simulink model "test_loadcase_pack_harness"  (R2026a)
settings: Solver=VariableStepAuto  StopTime=2000  AbsTol=1e-3
libraries: fl_lib x3, simulink x2, pack_5p48s8p_Thr_library x2, nesl_utility x2, pack_5p48s8p_1g10g1_5g1g5_Thr_library x1, pack_5p48s8p_1g10g1_Thr_library x1
Description:
  | Copyright 2023-2026 The MathWorks, Inc.
settings Model: Creator=smiller  LastModifiedBy=smiller
settings DebuggingCC: SymbolicDimsDataTypeCodeGenerationDiagnostic=none
settings SimscapeCC: SimscapeNominalValues="[{\"value\":\"1\",\"unit\":\"A\"},{\"value\":\"1\",\"unit\":\"bar\"},{\"value\":\"1\",\"unit\":\"cm^2\"},{\"value\":\"1\",\"unit\":\"cm^3/s\"},{\"value\":\"1\",\"unit\":\"kJ/kg\"},{\"value\":\"1\",\"unit\":\"kW\"},{\"value\":\"1\",\"unit\":\"l\"},{\"value\":\"1\",\"unit\":\"N\"},{\"value\":\"1\",\"unit\":\"N*m\"},{\"value\":\"1\",\"unit\":\"V\"}]"  SimscapeLogSimulationStatistics=on  SimscapeLogName=simlog_test_loadcase_pack

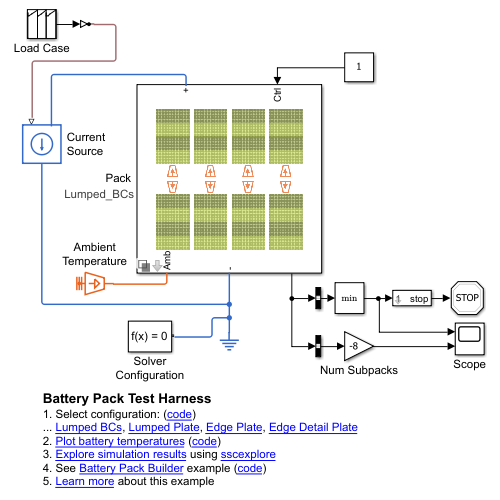
[thumbnail: Simulink's stored preview of the top-level diagram]
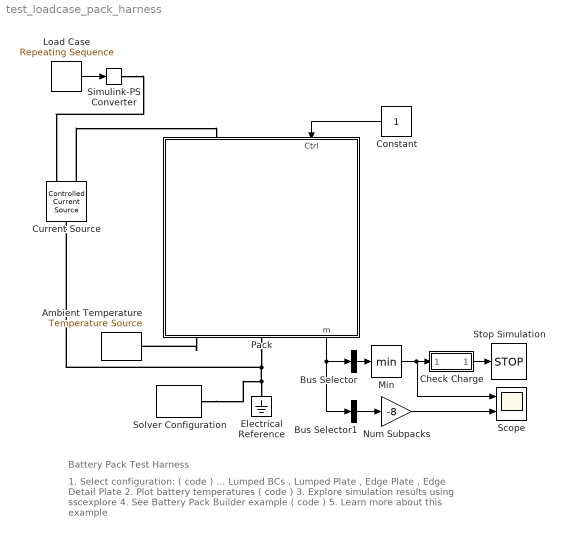
== system test_loadcase_pack_harness ==
  note: 1. Select configuration: ( code )
      | ... Lumped BCs , Lumped Plate , Edge Plate , Edge Detail Plate
      | 2. Plot battery temperatures ( code )
      | 3. Explore simulation results using sscexplore
      | 4. See Battery Pack Builder example ( code )
      | 5. Learn more about this example
  note: Battery Pack Test Harness
  Ambient Temperature : fl_lib/Thermal/Thermal Sources/Temperature Source  temperature=298 K
  Bus Selector : BusSelector  OutputSignals=A1.socC.M1  OutputAsBus=on
  Bus Selector1 : BusSelector  OutputSignals=A1.i.M1  OutputAsBus=on
  Check Charge : Subsystem  mask{q_battery_limit=0.3}
      mask prompts: q_battery_limit "Battery charge lower limit (A*hr)"
  Constant : Constant
  Current Source : fl_lib/Electrical/Electrical Sources/Controlled Current Source
  Electrical Reference : fl_lib/Electrical/Electrical Elements/Electrical Reference
  Load Case : simulink/Sources/Repeating Sequence  rep_seq_t="[0 1   2    32  33 300 800 2000]"  rep_seq_y=[0 0 450 450 400 400 440 510]
  Min : MinMax
  Num Subpacks : Gain  Gain=-8
  Pack : Subsystem  Variant=on  VariantControlMode=label  VariantControl=Choice  LabelModeActiveChoice=Lumped_BCs
      settings: AttributesFormatString=%<LabelModeActiveChoice>  PortSchema="{\"entries\":[{\"content\":{\"sides\":[{\"content\":{\"connectorIds\":[]},\"type\":\"ConnectorPlacement.EquallySpacedRectSide\",\"uuid\":\"bec220b6-5387-4603-a5dd-35505306a8ba\"},{\"content\":{\"connectorIds\":[],\"side\":\"RIGHT\"},\"type\":\"ConnectorPlacement.EquallySpacedRectSide\",\"uuid\":\"5cb410c8-66f5-4af1-8039-25d6dadf8cb5\"},{\"content\":{\"connectorIds\":[\"In1\",\"LConn1\"],\"side\":\"TOP\"},\"type\":\"ConnectorPlacement.EquallySpacedRectSide\",\"uuid\":\"ed36041a-2d53-45b1-8345-974004737ecd\"},{\"content\":{\"connectorIds\":[\"Out1\",\"RConn1\",\"RConn2\"],\"side\":\"BOTTOM\"},\"type\":\"ConnectorPlacement.EquallySpacedRectSide\",\"uuid\":\"d08fb284-6cdb-48c8-9fc2-d155432acf5d\"}]},\"type\":\"ConnectorPlacement.EquallySpacedConnector\",\"uuid\":\"570f951f-0a17-4653-8d49-20793e9a5a68\"}],\"packageUris\":[\"http://schema.mathworks.com/mf0/Connector/R2020b\"],\"version\":\"1.0\"}"
  Scope : Scope  NumInputPorts=2
      settings: Title=Battery SOC  ActiveDisplayYMinimum=0.2125  ActiveDisplayYMaximum=1.0875
  Simulink-PS Converter : nesl_utility/Simulink-PS Converter  PhysicalDomain=network_engine_domain  SubClassName=ps_input  LeftPortType=input  RightPortType=output  PseudoPeriodic=off  Frequencies=[]  NoiseDistribution=none  NoiseParameters=[]  Unit=1  AffineConversion=off  FilteringAndDerivatives=filter  SimscapeFilterOrder=1  InputFilterTimeConstant=0.01  UdotUserProvided=0
  Solver Configuration : nesl_utility/Solver Configuration  PhysicalDomain=network_engine_domain  SubClassName=solver  LeftPortType=input  RightPortType=generic  Tones=[]  Harmonics=[]  SimulateNoise=off  Profile=off  UseLocalSampling=off  EnableSwitchedLinearOptims=on  FrequencyDomain=off  UseCCode=off  RelTol=0.001  AbsTol=1e-06  MinStep=1e-09  ToWorkspace=off  RevertToSquareIcSolve=off  NumHomotopyIterations=100  PhasorMode=off  PhasorModeNumHarmonics=1  ConsistencySolver=NEWTON_XTOL_AFTER_FTOL  CanonicalOrdering=UNORDERED  OptimizeIntermediates=UNOPTIMIZED  IndexReductionMethod=None  DoDC=off  ResidualTolerance=1e-09  ConsistencyTolSource=GLOBAL  ConsistencyAbsTol=0.001  ConsistencyRelTol=0.001  ConsistencyTolFactor=0.001  UseLocalSolver=off  LocalSolverChoice=NE_BACKWARD_EULER_ADVANCER  ResolveIndetEquations=on  FunctionEvalNumThread=1  LocalSolverSampleTime=0.001  DoFixedCost=off  MaxNonlinIter=3  MaxModeIter=2  ComputeImpulses=off  ImpulseIterations=2  LinearAlgebra=auto  LinearAlgebraNumThread=0  EquationFormulation=NE_TIME_EF  DelaysMemoryBudget=1024  AutomaticFiltering=on  FilteringTimeConstant=0.001  PartitionStorageMethod=AS_NEEDED  PartitionMemoryBudget=1024  PartitionMethod=ROBUST  MultibodyUseLocalSolver=off  MultibodyLocalSolverChoice=ODE1  MultibodyLocalSolverSampleTime=0.001
  Stop Simulation : Stop
  wires:
  Min/1 -> Scope/1, Check Charge/1(In1)
  Check Charge/1(stop) -> Stop Simulation/1
  Load Case/1 -> Simulink-PS Converter/1
  Bus Selector1/1 -> Num Subpacks/1
  Bus Selector/1 -> Min/1
  Constant/1 -> Pack/1(Ctrl)
  Pack/1(m) -> Bus Selector/1, Bus Selector1/1
  Num Subpacks/1 -> Scope/2
  connections:
  Simulink-PS Converter/RConn1 -- Current Source/RConn1
  Solver Configuration/RConn1 -- Electrical Reference/LConn1 -- Current Source/LConn1 -- Pack/RConn1
  Current Source/RConn2 -- Pack/LConn1
  Pack/RConn2 -- Ambient Temperature/LConn1

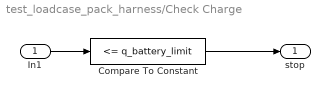
== system test_loadcase_pack_harness/Check Charge ==
  In1 : Inport
  Compare To Constant : simulink/Logic and Bit Operations/Compare To Constant  relop=<=  const=q_battery_limit  OutDataTypeStr=boolean
  stop : Outport  VectorParamsAs1DForOutWhenUnconnected=off
  wires:
  Compare To Constant/1 -> stop/1
  In1/1 -> Compare To Constant/1

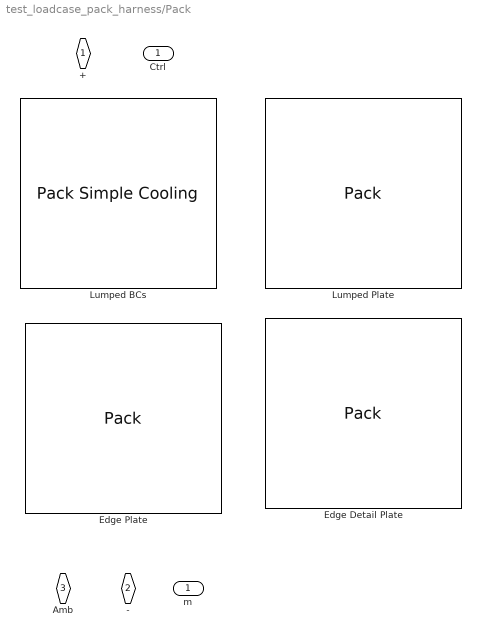
== system test_loadcase_pack_harness/Pack ==
  Ctrl : Inport
  Edge Detail Plate : pack_5p48s8p_1g10g1_5g1g5_Thr_library/Pack  VariantControl=Edge_Detail_Plate  cell_param=ModuleType1  targets=targets_5p48s8p_1g10g1_5g1g5_thr  plate=plate_5p48s_1g10g1_5g1g5_thr  batt_obj=batt_5p48s_1g10g1_5g1g5_thr
  Edge Plate : pack_5p48s8p_1g10g1_Thr_library/Pack  VariantControl=Edge_Plate  cell_param=ModuleType1  targets=targets_5p48s8p_1g10g1_thr  plate=plate_5p48s_1g10g1_thr  batt_obj=batt_5p48s_1g10g1_thr
  Lumped BCs : pack_5p48s8p_Thr_library/Pack Simple Cooling  VariantControl=Lumped_BCs  cell_param=ModuleType1  targets=targets_5p48s8p_thr  batt_obj=batt_5p48s_thr  coolant_temp=[23 26]
  Lumped Plate : pack_5p48s8p_Thr_library/Pack  VariantControl=Lumped_Plate  cell_param=ModuleType1  targets=targets_5p48s8p_thr  plate=plate_5p48s_thr  batt_obj=batt_5p48s_thr
  + : PMIOPort  Side=Left
  - : PMIOPort  Port=2  Side=Right
  Amb : PMIOPort  Port=3  Side=Right
  m : Outport
